simulink model "M2_motor_load"  (Simulink 10.2)
settings: Solver=ode4  StartTime=0.0  StopTime=3  FixedStep=T_s  RelTol=1e-3
InitFcn:
  | init
undefined symbols (not defined in the file): A_v, b_l, b_m, b_v, J_l, J_m, k, L, omega_v, R, theta_0, V_bar
settings Model: Creator=ioannis  LastModifiedBy=michelefocchi
settings DataIOCC: SaveFormat=Dataset  SignalLoggingSaveFormat=Dataset
settings OptimizationCC: LifeSpan=auto
settings DebuggingCC: UnderspecifiedInitializationDetection=Simplified  MergeDetectMultiDrivingBlocksExec=error  FcnCallInpInsideContextMsg=error  SFUnexpectedBacktrackingDiag=error  SFNoUnconditionalDefaultTransitionDiag=error  SFExecutionAtInitializationDiag=warning
settings HardwareCC: ProdBitPerPointer=64  ProdBitPerSizeT=64  ProdBitPerPtrDiffT=64  ProdLargestAtomicFloat=Float  ProdIntDivRoundTo=Zero  ProdEndianess=LittleEndian  ProdWordSize=64  ProdHWDeviceType=Intel->x86-64 (Windows64)
settings ModelReferenceCC: PropagateSignalLabelsOutOfModel=on
settings SFSimCC: SimUseLocalCustomCode=on
settings RTWCC: RTWUseLocalCustomCode=on
settings CodeAppCC: StateflowObjectComments=off
settings GRTTargetCC: TargetLangStandard=C99 (ISO)  CombineOutputUpdateFcns=on  GRTInterface=off
settings ConfigComp: CovMetricSettings=dwe  CovSaveCumulativeToWorkspaceVar=off  CovSaveSingleToWorkspaceVar=off  CovExternalEMLEnable=on

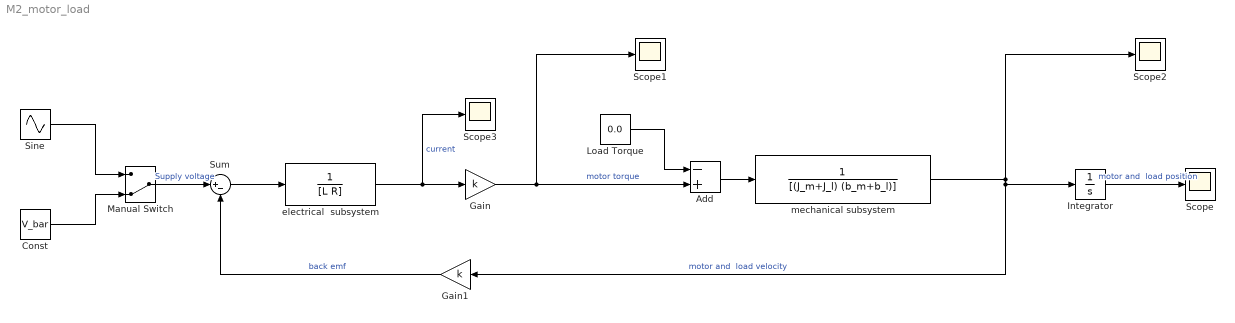
== system M2_motor_load ==
  Add : Sum  Inputs=-+
  "Const " : Constant  Value=V_bar
  Gain : Gain  Gain=k
  Gain1 : Gain  Gain=k
  Integrator : Integrator  InitialCondition=theta_0
  Load Torque : Constant  Value=0.0
  Manual Switch : ManualSwitch  CurrentSetting=0
  Scope{,1..3} (4 alike) : Scope
  "Sine " : Sin  Amplitude=A_v  Bias=b_v  Frequency=omega_v  SampleTime=0
  Sum : Sum  Inputs=|+-
  electrical  subsystem : TransferFcn  Denominator=[L R]
  mechanical subsystem : TransferFcn  Denominator=[(J_m+J_l) (b_m+b_l)]
  wires:
  Gain/1 -> Scope1/1, Add/2  "motor torque"
  mechanical subsystem/1 -> Gain1/1, Integrator/1, Scope2/1  "motor and  load velocity"
  Sum/1 -> electrical  subsystem/1
  Gain1/1 -> Sum/2  "back emf"
  Integrator/1 -> Scope/1  "motor and  load position"
  electrical  subsystem/1 -> Scope3/1, Gain/1  "current"
  "Sine "/1 -> Manual Switch/1
  "Const "/1 -> Manual Switch/2
  Manual Switch/1 -> Sum/1  "Supply voltage"
  Add/1 -> mechanical subsystem/1
  Load Torque/1 -> Add/1
